simulink model "SimulinkProportionalComponent"  (R2023a)
settings: Solver=VariableStepAuto  StartTime=0.0  StopTime=100  RelTol=1e-3
undefined symbols (not defined in the file or in its folder): freq
settings Model: Creator=Lenovo  LastModifiedBy=17634948724

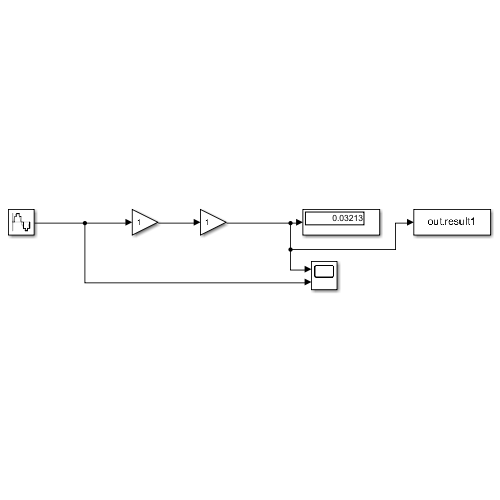
[thumbnail: Simulink's stored preview of the top-level diagram]
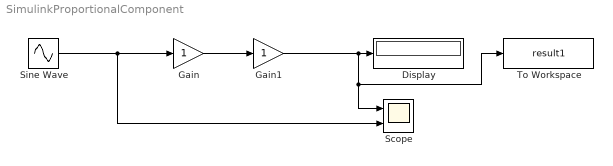
== system SimulinkProportionalComponent ==
  Display : Display
  Gain : Gain
  Gain1 : Gain
  Scope : Scope  NumInputPorts=2
  Sine Wave : Sin  Amplitude=length  Frequency=freq  SampleTime=0.1
  To Workspace : ToWorkspace  VariableName=result1  SaveFormat=Timeseries  SampleTime=-1
  wires:
  Sine Wave/1 -> Scope/2, Gain/1
  Gain/1 -> Gain1/1
  Gain1/1 -> To Workspace/1, Scope/1, Display/1
